simulink model "switch_case"  (R2014a)
settings: Solver=FixedStepDiscrete  StartTime=0.0  StopTime=10.0  FixedStep=0.1  RelTol=1e-3
settings Model: BufferReuse=off  Creator=yoshi12  LastModifiedBy=ts1413
settings OptimizationCC: BlockReduction=off  OptimizeBlockIOStorage=off  BufferReuse=off  GlobalBufferReuse=off  ExpressionFolding=off  LocalBlockOutputs=off  OptimizeModelRefInitCode=on  LifeSpan=1
settings RTWCC: SystemTargetFile=ert.tlc  GenCodeOnly=on  TemplateMakefile=ert_default_tmf  Description=Embedded Coder  ProcessScript=ert_make_rtw_hook
settings CodeAppCC: IgnoreCustomStorageClasses=off
settings ERTTargetCC: ParMdlRefBuildCompliant=on  CompOptLevelCompliant=on  ConcurrentExecutionCompliant=on  ERTFirstTimeCompliant=on  ModelStepFunctionPrototypeControlCompliant=on  CPPClassGenCompliant=on  InlinedParameterPlacement=Hierarchical  ERTCustomFileTemplate=example_file_process.tlc

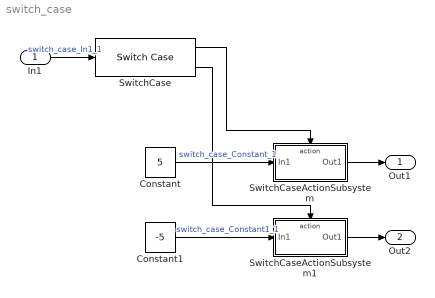
== system switch_case ==
  In1 : Inport
  Constant : Constant  Value=5
  Constant1 : Constant  Value=-5
  SwitchCase : SwitchCase
  SwitchCaseActionSubsystem : Subsystem  TreatAsAtomicUnit=on
  SwitchCaseActionSubsystem1 : Subsystem  TreatAsAtomicUnit=on
  Out1 : Outport
  Out2 : Outport  Port=2
  wires:
  In1/1 -> SwitchCase/1  "switch_case_In1_1"
  SwitchCase/1 -> SwitchCaseActionSubsystem/Action
  SwitchCase/2 -> SwitchCaseActionSubsystem1/Action
  SwitchCaseActionSubsystem/1(Out1) -> Out1/1
  SwitchCaseActionSubsystem1/1(Out1) -> Out2/1
  Constant/1 -> SwitchCaseActionSubsystem/1(In1)  "switch_case_Constant_1"
  Constant1/1 -> SwitchCaseActionSubsystem1/1(In1)  "switch_case_Constant1_1"

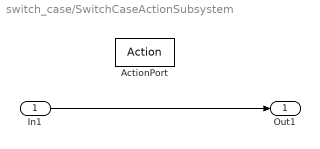
== system switch_case/SwitchCaseActionSubsystem ==
  In1 : Inport
  ActionPort : ActionPort  ActionType=case
  Out1 : Outport
  wires:
  In1/1 -> Out1/1

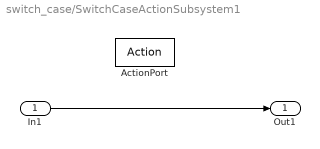
== system switch_case/SwitchCaseActionSubsystem1 ==
  In1 : Inport
  ActionPort : ActionPort  ActionType=default
  Out1 : Outport
  wires:
  In1/1 -> Out1/1
